simulink model "Simple_4Quad_payload_10_2017a"  (R2017a)
settings: Solver=ode45  StartTime=0.0  StopTime=100  FixedStep=0.001  RelTol=1e-3
InitFcn:
  | Simple_4Quad_payload_10_const
values from neighbouring files (symbols this model uses):
  All_rho = [d1 0 0 ... (first row only)    [Colab_4Quad_model_01_const.m]    (also in Colab_4Quad_model_02_const.m; Simple_4Quad_payload_04_const.m; Simple_4Quad_payload_05_const.m; Simple_4Quad_payload_06_const.m)
  alpha_chatt = 0.1    [Simple_4Quad_payload_09_const.m]    (also in Simple_4Quad_payload_10_const.m = 0.001; Simple_4Quad_payload_11_const.m = 0.01; Simple_4Quad_payload_12_const.m = 0.01)
  alphaTF = 0.1    [Simple_4Quad_payload_08_const.m]    (also in Simple_4Quad_payload_09_const.m = 0.5; Simple_4Quad_payload_10_const.m = 1; Simple_4Quad_payload_11_const.m = 0.5; Simple_4Quad_payload_12_const.m = 10)
  B_ob = [zeros(3);eye(3)]    [Simple_4Quad_payload_04_const.m]    (also in Simple_4Quad_payload_05_const.m; Simple_4Quad_payload_06_const.m; Simple_4Quad_payload_07_const.m; Simple_4Quad_payload_08_const.m)
  BBT_inv = ((B'*B)^(-1))*B'    [Simple_2Quad_payload_03_const.m]    (also in Simple_4Quad_payload_04_const.m = ((BR'*BR)^(-1))*BR'; Simple_4Quad_payload_05_const.m = ((BR'*BR)^(-1))*BR'; Simple_4Quad_payload_06_const.m = ((BR'*BR)^(-1))*BR'; Simple_4Quad_payload_07_const.m = ((BR'*BR)^(-1))*BR')
  BBT_invp = ((BRp'*BRp)^(-1))*BRp'    [Simple_4Quad_payload_10_const.m]    (also in Simple_4Quad_payload_11_const.m; Simple_4Quad_payload_12_const.m)
  BR = 1e0*eye(n)    [Simple_4Quad_payload_04_const.m]    (also in Simple_4Quad_payload_05_const.m; Simple_4Quad_payload_06_const.m; Simple_4Quad_payload_07_const.m; Simple_4Quad_payload_08_const.m)
  BRp = 1e0*eye(np)    [Simple_4Quad_payload_10_const.m]    (also in Simple_4Quad_payload_11_const.m; Simple_4Quad_payload_12_const.m)
  C_ob = [eye(3) zeros(3)]    [Simple_4Quad_payload_04_const.m]    (also in Simple_4Quad_payload_05_const.m; Simple_4Quad_payload_06_const.m; Simple_4Quad_payload_07_const.m; Simple_4Quad_payload_08_const.m)
  cons_sld = 0.001    [Simple_4Quad_payload_10_const.m]    (also in Simple_4Quad_payload_11_const.m = 0.01; Simple_4Quad_payload_12_const.m = 0.01)
  d1 = 0.25    [Colab_4Quad_model_01_const.m]    (also in Colab_4Quad_model_02_const.m = 0.5; Simple_4Quad_payload_01_const.m = 1; Simple_4Quad_payload_02_const.m = 1; Simple_4Quad_payload_03_const.m = 1)
  d2 = 0.25    [Colab_4Quad_model_01_const.m]    (also in Colab_4Quad_model_02_const.m = 0.5; Simple_4Quad_payload_01_const.m = 1; Simple_4Quad_payload_02_const.m = 1; Simple_4Quad_payload_03_const.m = 1)
  Des_rel_dist = 2    [Simple_4Quad_payload_01_const.m]    (also in Simple_4Quad_payload_02_const.m = 4; Simple_4Quad_payload_03_const.m = 4; Simple_4Quad_payload_04_const.m; Simple_4Quad_payload_05_const.m)
  g = 9.81    [Colab_4Quad_model_01_const.m]    (also in Colab_4Quad_model_02_const.m; Simple_2Quad_payload_01_const.m; Simple_2Quad_payload_02_const.m; Simple_2Quad_payload_03_const.m)
  gamma_0 = 1e-0*diag([1e-3;1e-0])    [Simple_2Quad_payload_03_const.m]    (also in Simple_4Quad_payload_04_const.m = 1e-0*diag([1e-6*ones(3,1);1e-0*ones(3,1)]); Simple_4Quad_payload_05_const.m = 1e-1*diag([1e-6*ones(3,1);1e-0*ones(3,1)]); Simple_4Quad_payload_06_const.m = 1e-0*diag([1e-6*ones(3,1);1e-0*ones(3,1)]); Simple_4Quad_payload_07_const.m = 1e-0*diag([1e-6*ones(3,1);1e-0*ones(3,1)]))
  gamma_0a = 1e-0*diag(1e-0*ones(3,1))    [Simple_4Quad_payload_10_const.m]    (also in Simple_4Quad_payload_11_const.m = 1e-0*diag(1e-6*ones(3,1)))
  gamma_0L = 1e-0*diag([1e-6*ones(3,1);1e-0*ones(3,1)])    [Simple_4Quad_payload_08_const.m]    (also in Simple_4Quad_payload_09_const.m; Simple_4Quad_payload_10_const.m = 1e+0*diag([1e-3*ones(3,1);1e-3*ones(3,1)]); Simple_4Quad_payload_11_const.m = 1e+0*diag([1e-3*ones(3,1);1e-3*ones(3,1)]); Simple_4Quad_payload_12_const.m = 1e+2*diag(1e-4*ones(3,1)))
  gamma_0p = 1e-0*diag(1e-3*ones(3,1))    [Simple_4Quad_payload_10_const.m]    (also in Simple_4Quad_payload_11_const.m = 1e-0*diag(1e-6*ones(3,1)))
  gamma_0r = 1e-0*diag(1e-3*ones(3,1))    [Simple_4Quad_payload_10_const.m]    (also in Simple_4Quad_payload_11_const.m = 1e-0*diag(1e-6*ones(3,1)); Simple_4Quad_payload_12_const.m = 1e+3*diag(1e-0*ones(3,1)))
  gamma_0v = 1e-0*diag([1e-0*ones(3,1);1e-0*ones(3,1)])    [Simple_4Quad_payload_08_const.m]    (also in Simple_4Quad_payload_09_const.m = 1e-0*diag([1e-6*ones(3,1);1e-6*ones(3,1)]); Simple_4Quad_payload_10_const.m = 1e+0*diag(1e-0*ones(3,1)); Simple_4Quad_payload_11_const.m = 1e+0*diag(1e-0*ones(3,1)); Simple_4Quad_payload_12_const.m = 1e+3*diag(1e-0*ones(3,1)))
  gamma_1 = 1e+2*diag([1e-3;1e-0])    [Simple_2Quad_payload_03_const.m]    (also in Simple_4Quad_payload_04_const.m = 1e+2*diag([1e-6*ones(3,1);1e-0*ones(3,1)]); Simple_4Quad_payload_05_const.m = 1e+2*diag([1e-6*ones(3,1);1e-0*ones(3,1)]); Simple_4Quad_payload_06_const.m = 1e+3*diag([1e-6*ones(3,1);1e-0*ones(3,1)]); Simple_4Quad_payload_07_const.m = 1e+3*diag([1e-6*ones(3,1);1e-0*ones(3,1)]))
  gamma_1a = 1e+0*diag(1e-0*ones(3,1))    [Simple_4Quad_payload_10_const.m]    (also in Simple_4Quad_payload_11_const.m = 1e+0*diag(1e-6*ones(3,1)))
  gamma_1L = 1e+3*diag([1e-6*ones(3,1);1e-0*ones(3,1)])    [Simple_4Quad_payload_08_const.m]    (also in Simple_4Quad_payload_09_const.m = 1e+2*diag([1e-6*ones(3,1);1e-0*ones(3,1)]); Simple_4Quad_payload_10_const.m = 1e+1*diag([1e-3*ones(3,1);1e-3*ones(3,1)]); Simple_4Quad_payload_11_const.m = 1e+0*diag([1e-3*ones(3,1);1e-3*ones(3,1)]); Simple_4Quad_payload_12_const.m = 1e+2*diag(1e-4*ones(3,1)))
  gamma_1p = 1e+0*diag(1e-3*ones(3,1))    [Simple_4Quad_payload_10_const.m]    (also in Simple_4Quad_payload_11_const.m = 1e+0*diag(1e-6*ones(3,1)))
  gamma_1r = 1e+0*diag(1e-3*ones(3,1))    [Simple_4Quad_payload_10_const.m]    (also in Simple_4Quad_payload_11_const.m = 1e+0*diag(1e-6*ones(3,1)); Simple_4Quad_payload_12_const.m = 1e+3*diag(1e-0*ones(3,1)))
  gamma_1v = 1e+3*diag([1e-0*ones(3,1);1e-0*ones(3,1)])    [Simple_4Quad_payload_08_const.m]    (also in Simple_4Quad_payload_09_const.m = 1e+2*diag([1e-6*ones(3,1);1e-6*ones(3,1)]); Simple_4Quad_payload_10_const.m = 1e+0*diag(1e-0*ones(3,1)); Simple_4Quad_payload_11_const.m = 1e+0*diag(1e-0*ones(3,1)); Simple_4Quad_payload_12_const.m = 1e+3*diag(1e-0*ones(3,1)))
  Ix = 0.166667    [Colab_4Quad_model_01_const.m]    (also in Colab_4Quad_model_02_const.m = 0.02; Simple_4Quad_payload_01_const.m = 1; Simple_4Quad_payload_02_const.m = 1; Simple_4Quad_payload_03_const.m = 1)
  Iy = 0.166667    [Colab_4Quad_model_01_const.m]    (also in Colab_4Quad_model_02_const.m = 0.02; Simple_4Quad_payload_01_const.m = 1; Simple_4Quad_payload_02_const.m = 1; Simple_4Quad_payload_03_const.m = 1)
  Iz = 0.166667    [Colab_4Quad_model_01_const.m]    (also in Colab_4Quad_model_02_const.m = 0.02; Simple_4Quad_payload_01_const.m = 1; Simple_4Quad_payload_02_const.m = 1; Simple_4Quad_payload_03_const.m = 1)
  Jo = diag([Ix;Iy;Iz])    [Colab_4Quad_model_01_const.m]    (also in Colab_4Quad_model_02_const.m; Simple_4Quad_payload_04_const.m; Simple_4Quad_payload_05_const.m; Simple_4Quad_payload_06_const.m)
  Jq = diag([0.0291 0.0291 0.0552])    [Colab_4Quad_model_01_const.m]    (also in Colab_4Quad_model_02_const.m = diag([0.03 0.03 0.06]); Simple_4Quad_payload_03_const.m = 1.2416e-3 * diag([1 1 2]); Simple_4Quad_payload_04_const.m = 1 * diag([1 1 2]); Simple_4Quad_payload_05_const.m = 1 * diag([1 1 2]))
  k1 = 1    [Simple_2Quad_payload_03_const.m]    (also in Simple_4Quad_payload_04_const.m; Simple_4Quad_payload_05_const.m; Simple_4Quad_payload_06_const.m; Simple_4Quad_payload_07_const.m)
  k2 = 0.1    [Simple_2Quad_payload_03_const.m]    (also in Simple_4Quad_payload_04_const.m; Simple_4Quad_payload_05_const.m; Simple_4Quad_payload_06_const.m; Simple_4Quad_payload_07_const.m)
  l = 3.1819    [Colab_4Quad_model_01_const.m]    (also in Colab_4Quad_model_02_const.m = 3; Simple_2Quad_payload_04_const.m = 1; Simple_4Quad_payload_01_const.m = 1; Simple_4Quad_payload_02_const.m = 2)
  m = 1.5    [Colab_4Quad_model_01_const.m]    (also in Colab_4Quad_model_02_const.m; Simple_2Quad_payload_04_const.m = 1; Simple_4Quad_payload_01_const.m = 1; Simple_4Quad_payload_02_const.m = 1)
  M = 1.0    (= 1)    [Colab_4Quad_model_01_const.m]    (also in Colab_4Quad_model_02_const.m; Simple_2Quad_payload_01_const.m; Simple_2Quad_payload_02_const.m; Simple_2Quad_payload_03_const.m)
  n = 2    [Simple_2Quad_payload_03_const.m]    (also in Simple_4Quad_payload_03_const.m = 6; Simple_4Quad_payload_04_const.m = 6; Simple_4Quad_payload_05_const.m = 6; Simple_4Quad_payload_06_const.m = 6)
  noise_var_RelAcc = 0e-6    (= 0)    [Simple_4Quad_payload_07_const.m]    (also in Simple_4Quad_payload_08_const.m; Simple_4Quad_payload_09_const.m; Simple_4Quad_payload_10_const.m; Simple_4Quad_payload_11_const.m)
  noise_var_RelPos = 0e-6    (= 0)    [Simple_4Quad_payload_07_const.m]    (also in Simple_4Quad_payload_08_const.m; Simple_4Quad_payload_09_const.m; Simple_4Quad_payload_10_const.m; Simple_4Quad_payload_11_const.m)
  np = 3    [Simple_4Quad_payload_10_const.m]    (also in Simple_4Quad_payload_11_const.m; Simple_4Quad_payload_12_const.m; constant_CAMFC2_Quad_New_02_Payload_01.m = 6)
  Q_ob = var_u_ob * eye(6)    [Simple_4Quad_payload_04_const.m]    (also in Simple_4Quad_payload_05_const.m; Simple_4Quad_payload_06_const.m; Simple_4Quad_payload_07_const.m; Simple_4Quad_payload_08_const.m)
  Qa = 1e-0*eye(np)    [Simple_4Quad_payload_10_const.m]    (also in Simple_4Quad_payload_11_const.m)
  QL = 1e-0*eye(n)    [Simple_4Quad_payload_08_const.m]    (also in Simple_4Quad_payload_09_const.m; Simple_4Quad_payload_10_const.m; Simple_4Quad_payload_11_const.m = 1e-2*eye(n); Simple_4Quad_payload_12_const.m = 1e-0*eye(np))
  Qp = 1e-0*eye(np)    [Simple_4Quad_payload_10_const.m]    (also in Simple_4Quad_payload_11_const.m = 1e-2*eye(np))
  QR = 1e-0*eye(n)    [Simple_4Quad_payload_04_const.m]    (also in Simple_4Quad_payload_05_const.m = 1e-1*eye(n); Simple_4Quad_payload_06_const.m; Simple_4Quad_payload_07_const.m; Simple_4Quad_payload_08_const.m)
  Qr = 1e-0*eye(np)    [Simple_4Quad_payload_10_const.m]    (also in Simple_4Quad_payload_11_const.m; Simple_4Quad_payload_12_const.m)
  Qv = 1e-0*eye(n)    [Simple_4Quad_payload_08_const.m]    (also in Simple_4Quad_payload_09_const.m; Simple_4Quad_payload_10_const.m = 1e-0*eye(np); Simple_4Quad_payload_11_const.m = 1e-2*eye(np); Simple_4Quad_payload_12_const.m = 1e-0*eye(np))
  R = 1e+0*eye(n)    [Simple_2Quad_payload_03_const.m]    (also in Simple_4Quad_payload_04_const.m = 1e+0*eye(m); Simple_4Quad_payload_05_const.m = 1e+0*eye(m); Simple_4Quad_payload_06_const.m; Simple_4Quad_payload_07_const.m)
  R_ob = var_y_ob * eye(3)    [Simple_4Quad_payload_04_const.m]    (also in Simple_4Quad_payload_05_const.m; Simple_4Quad_payload_06_const.m; Simple_4Quad_payload_07_const.m; Simple_4Quad_payload_08_const.m)
  rho_0 = 1e-0    (= 1)    [Simple_2Quad_payload_03_const.m]    (also in Simple_4Quad_payload_04_const.m; Simple_4Quad_payload_05_const.m = 0.1; Simple_4Quad_payload_06_const.m; Simple_4Quad_payload_07_const.m)
  rho_0a = 1e-0    (= 1)    [Simple_4Quad_payload_10_const.m]    (also in Simple_4Quad_payload_11_const.m)
  rho_0L = 1e-0    (= 1)    [Simple_4Quad_payload_08_const.m]    (also in Simple_4Quad_payload_09_const.m; Simple_4Quad_payload_10_const.m; Simple_4Quad_payload_11_const.m; Simple_4Quad_payload_12_const.m)
  rho_0p = 1e-0    (= 1)    [Simple_4Quad_payload_10_const.m]    (also in Simple_4Quad_payload_11_const.m)
  rho_0r = 1e-0    (= 1)    [Simple_4Quad_payload_10_const.m]    (also in Simple_4Quad_payload_11_const.m; Simple_4Quad_payload_12_const.m = 0.001)
  rho_0v = 1e-1    (= 0.1)    [Simple_4Quad_payload_08_const.m]    (also in Simple_4Quad_payload_09_const.m = 1; Simple_4Quad_payload_10_const.m = 1; Simple_4Quad_payload_11_const.m = 1; Simple_4Quad_payload_12_const.m = 1)
  rho_1 = 1e-0    (= 1)    [Simple_2Quad_payload_03_const.m]    (also in Simple_4Quad_payload_04_const.m; Simple_4Quad_payload_05_const.m; Simple_4Quad_payload_06_const.m; Simple_4Quad_payload_07_const.m)
  rho_1a = 1e-0    (= 1)    [Simple_4Quad_payload_10_const.m]    (also in Simple_4Quad_payload_11_const.m)
  rho_1L = 1e-0    (= 1)    [Simple_4Quad_payload_08_const.m]    (also in Simple_4Quad_payload_09_const.m; Simple_4Quad_payload_10_const.m; Simple_4Quad_payload_11_const.m; Simple_4Quad_payload_12_const.m)
  rho_1p = 1e-0    (= 1)    [Simple_4Quad_payload_10_const.m]    (also in Simple_4Quad_payload_11_const.m)
  rho_1r = 1e-0    (= 1)    [Simple_4Quad_payload_10_const.m]    (also in Simple_4Quad_payload_11_const.m; Simple_4Quad_payload_12_const.m)
  rho_1v = 1e-0    (= 1)    [Simple_4Quad_payload_08_const.m]    (also in Simple_4Quad_payload_09_const.m; Simple_4Quad_payload_10_const.m; Simple_4Quad_payload_11_const.m; Simple_4Quad_payload_12_const.m)
  Rp = 1e+0*eye(np)    [Simple_4Quad_payload_10_const.m]    (also in Simple_4Quad_payload_11_const.m; Simple_4Quad_payload_12_const.m)
  xo_init = 0    [Simple_4Quad_payload_10_const.m]    (also in Simple_4Quad_payload_11_const.m; Simple_4Quad_payload_12_const.m)
  yo_init = 0    [Simple_4Quad_payload_10_const.m]    (also in Simple_4Quad_payload_11_const.m; Simple_4Quad_payload_12_const.m)
  zo_init = 0    [Simple_4Quad_payload_10_const.m]    (also in Simple_4Quad_payload_11_const.m; Simple_4Quad_payload_12_const.m)
libraries: simulink x2
(part 4 of 5)

== matlab function Simple_4Quad_payload_10_2017a/Controllers and Observers/Controller and Observer - Agent4/Rotational #4/Differentiator/Sliding differentiator ==
  data: u output; u1 input; e input; n parameter; k1 parameter; cons_sld parameter
function u = fcn(u1,e,n,k1,cons_sld)

b=k1;

ABS = zeros(n,1);
for i=1:n
    if e(i)>0
        ABS(i) = e(i);
    else
        ABS(i) = -e(i);
    end
end
SGN = e ./ (ABS + cons_sld);

u = u1 - b*(ABS.^0.5).*SGN;

end

== matlab function Simple_4Quad_payload_10_2017a/Controllers and Observers/Controller and Observer - Agent4/Rotational #4/Differentiator/Sliding differentiator1 ==
  data: Du1 output; e input; n parameter; k2 parameter; cons_sld parameter
function Du1 = fcn(e,n,k2,cons_sld)

a=k2;

ABS = zeros(n,1);
for i=1:n
    if e(i)>0
        ABS(i) = e(i);
    else
        ABS(i) = -e(i);
    end
end
SGN = e ./ (ABS + cons_sld);

Du1 = - a*SGN;

end

== matlab function Simple_4Quad_payload_10_2017a/Controllers and Observers/Controller and Observer - Agent4/Rotational #4/g-Estimator ==
  data: sigma input; g_hat input; P input; rho_1 parameter; gamma_1 parameter; Dg_hat output
function Dg_hat = fcn(sigma,g_hat,P,rho_1,gamma_1)

Dg_hat = - gamma_1 * P * sigma - rho_1 * gamma_1 * g_hat;

end

== matlab function Simple_4Quad_payload_10_2017a/Controllers and Observers/Controller and Observer - Agent4/Rotational #4/g-Estimator1 ==
  data: sigma input; x input; P input; rho_0 parameter; gamma_0 parameter; Da_hat output; a_hat input
function Da_hat = fcn(sigma,x,P,rho_0,gamma_0,a_hat)

DVa_hat = - gamma_0 * P * diag(sigma) * (x - sigma) - rho_0 * gamma_0 * diag(a_hat);

Da_hat = diag(DVa_hat);

end

== matlab function Simple_4Quad_payload_10_2017a/Controllers and Observers/Controller and Observer - Agent4/Rotational #4/main ==
  data: sigma input; zeta input; u output; Dy_d input; R parameter; P input; a_hat input; BR parameter; g_hat input; x input; QR parameter; BBT_inv parameter; n parameter
function u = fcn(sigma,zeta,Dy_d,R,P,a_hat,BR,g_hat,x,QR,BBT_inv,n)

u1 = (1/2) * R * BR' * P * sigma;
u2 = BBT_inv * (Dy_d - a_hat*x + (eye(n) + 2*(((P)^(-1)*QR)) + a_hat)*sigma - g_hat - zeta) - (3/4) * R * BR' * P * sigma;

u = u1 + u2;

end

== matlab function Simple_4Quad_payload_10_2017a/Controllers and Observers/Controller and Observer - Agent4/Rotational #4/variable change ==
  data: X input; Xd input; x_mod output; u input; xd_mod output; e_mod output
function [x_mod,xd_mod,e_mod] = fcn(X,Xd,u)

x_mod = X;

xd_mod = [Xd;u(1:3)];

e_mod = xd_mod - x_mod;


end

== matlab function Simple_4Quad_payload_10_2017a/Controllers and Observers/Controlelr and Observer - Agent3/Observer3/Kalman_Filter3 ==
  data: P_ob input; DP_ob output; xhat_ob input; Dxhat_ob output; Q_ob parameter; R_ob parameter; C_ob parameter; B_ob parameter; wo input; Dwo input; Rel_Posi_local input; Rel_Acci_local input; Agent_Num input; All_rho parameter; l parameter
function [DP_ob,Dxhat_ob] = fcn(P_ob,xhat_ob,Q_ob, R_ob, C_ob, B_ob,wo,Dwo,Rel_Posi_local,Rel_Acci_local,Agent_Num,All_rho,l)

rhoi = All_rho(Agent_Num,:)';

wo_skew = [...
    0 -wo(3) wo(2);
    wo(3) 0 -wo(1);
    -wo(2) wo(1) 0];

Dwo_skew = [...
    0 -Dwo(3) Dwo(2);
    Dwo(3) 0 -Dwo(1);
    -Dwo(2) Dwo(1) 0];

A1_ob = wo_skew * wo_skew + Dwo_skew;
A2_ob = 2*wo_skew;

A_ob = [zeros(3) eye(3);
    -A1_ob -A2_ob];

y_ob = (1/l) * ( Rel_Posi_local - rhoi );
u_ob = (1/l) * ( Rel_Acci_local - A1_ob*rhoi );

DP_ob = A_ob'*P_ob + P_ob*A_ob - P_ob*C_ob'*R_ob*C_ob*P_ob + Q_ob;
K_ob = P_ob * C_ob' * R_ob;
Dxhat_ob = A_ob*xhat_ob + B_ob*u_ob + K_ob*(y_ob - C_ob*xhat_ob);

end

== matlab function Simple_4Quad_payload_10_2017a/Controllers and Observers/Controlelr and Observer - Agent3/Observer3/Observer_Finalization3 ==
  data: xhati input; qhati output; Dqhati output
function [qhati,Dqhati] = fcn(xhati)

qhati = xhati(1:3);
Dqhati = xhati(4:6);

end

== matlab function Simple_4Quad_payload_10_2017a/Controllers and Observers/Controller and Observer - Agent4/Observer4/Kalman_Filter4 ==
  data: P_ob input; DP_ob output; xhat_ob input; Dxhat_ob output; Q_ob parameter; R_ob parameter; C_ob parameter; B_ob parameter; wo input; Dwo input; Rel_Posi_local input; Rel_Acci_local input; Agent_Num input; All_rho parameter; l parameter
function [DP_ob,Dxhat_ob] = fcn(P_ob,xhat_ob,Q_ob, R_ob, C_ob, B_ob,wo,Dwo,Rel_Posi_local,Rel_Acci_local,Agent_Num,All_rho,l)

rhoi = All_rho(Agent_Num,:)';

wo_skew = [...
    0 -wo(3) wo(2);
    wo(3) 0 -wo(1);
    -wo(2) wo(1) 0];

Dwo_skew = [...
    0 -Dwo(3) Dwo(2);
    Dwo(3) 0 -Dwo(1);
    -Dwo(2) Dwo(1) 0];

A1_ob = wo_skew * wo_skew + Dwo_skew;
A2_ob = 2*wo_skew;

A_ob = [zeros(3) eye(3);
    -A1_ob -A2_ob];

y_ob = (1/l) * ( Rel_Posi_local - rhoi );
u_ob = (1/l) * ( Rel_Acci_local - A1_ob*rhoi );

DP_ob = A_ob'*P_ob + P_ob*A_ob - P_ob*C_ob'*R_ob*C_ob*P_ob + Q_ob;
K_ob = P_ob * C_ob' * R_ob;
Dxhat_ob = A_ob*xhat_ob + B_ob*u_ob + K_ob*(y_ob - C_ob*xhat_ob);

end

== matlab function Simple_4Quad_payload_10_2017a/Controllers and Observers/Controller and Observer - Agent4/Observer4/Observer_Finalization4 ==
  data: xhati input; qhati output; Dqhati output
function [qhati,Dqhati] = fcn(xhati)

qhati = xhati(1:3);
Dqhati = xhati(4:6);

end

== matlab function Simple_4Quad_payload_10_2017a/Relative measurements/Relative position measurements in payload local frame ==
  data: PHI input; Rel_Pos_local1 output; ro input; r1 input; r2 input; r3 input; r4 input; Rel_Pos_local2 output; Rel_Pos_local3 output; Rel_Pos_local4 output
function [Rel_Pos_local1,Rel_Pos_local2,Rel_Pos_local3,Rel_Pos_local4] = fcn(PHI,ro,r1,r2,r3,r4)

phi = PHI(1);
theta = PHI(2);
psi = PHI(3);

Ro = [cos(psi)*cos(theta) cos(psi)*sin(theta)*sin(phi)-sin(psi)*cos(phi) cos(psi)*sin(theta)*cos(phi)+sin(psi)*sin(phi);
    sin(psi)*cos(theta) sin(psi)*sin(theta)*sin(phi)+cos(psi)*cos(phi) sin(psi)*sin(theta)*cos(phi)-cos(psi)*sin(phi);
    -sin(theta) cos(theta)*sin(phi) cos(theta)*cos(phi)];

Rel_Pos_local1 = Ro' * (r1 - ro);
Rel_Pos_local2 = Ro' * (r2 - ro);
Rel_Pos_local3 = Ro' * (r3 - ro);
Rel_Pos_local4 = Ro' * (r4 - ro);

end

== matlab function Simple_4Quad_payload_10_2017a/Dynamic model of the entire system/Drone absolute position computation ==
  data: q1 input; r1 output; r2 output; r3 output; r4 output; q2 input; q3 input; q4 input; All_rho parameter; l parameter; ro input; PHI input
function [r1,r2,r3,r4] = fcn(q1,q2,q3,q4,All_rho, l,ro,PHI)

rho1 = All_rho(1,:)';
rho2 = All_rho(2,:)';
rho3 = All_rho(3,:)';
rho4 = All_rho(4,:)';

phi = PHI(1);
theta = PHI(2);
psi = PHI(3);

Ro = [cos(psi)*cos(theta) cos(psi)*sin(theta)*sin(phi)-sin(psi)*cos(phi) cos(psi)*sin(theta)*cos(phi)+sin(psi)*sin(phi);
    sin(psi)*cos(theta) sin(psi)*sin(theta)*sin(phi)+cos(psi)*cos(phi) sin(psi)*sin(theta)*cos(phi)-cos(psi)*sin(phi);
    -sin(theta) cos(theta)*sin(phi) cos(theta)*cos(phi)];

r1 = ro + Ro*rho1 - l*q1;
r2 = ro + Ro*rho2 - l*q2;
r3 = ro + Ro*rho3 - l*q3;
r4 = ro + Ro*rho4 - l*q4;

end

== matlab function Simple_4Quad_payload_10_2017a/Relative measurements/Relative acceleration measurements in payload local frame ==
  data: PHI input; Rel_Acc_local1 output; DDro input; DDr1 input; DDr2 input; DDr3 input; DDr4 input; Rel_Acc_local2 output; Rel_Acc_local3 output; Rel_Acc_local4 output
function [Rel_Acc_local1,Rel_Acc_local2,Rel_Acc_local3,Rel_Acc_local4] = fcn(PHI,DDro,DDr1,DDr2,DDr3,DDr4)

phi = PHI(1);
theta = PHI(2);
psi = PHI(3);

Ro = [cos(psi)*cos(theta) cos(psi)*sin(theta)*sin(phi)-sin(psi)*cos(phi) cos(psi)*sin(theta)*cos(phi)+sin(psi)*sin(phi);
    sin(psi)*cos(theta) sin(psi)*sin(theta)*sin(phi)+cos(psi)*cos(phi) sin(psi)*sin(theta)*cos(phi)-cos(psi)*sin(phi);
    -sin(theta) cos(theta)*sin(phi) cos(theta)*cos(phi)];

Rel_Acc_local1 = Ro' * (DDr1 - DDro);
Rel_Acc_local2 = Ro' * (DDr2 - DDro);
Rel_Acc_local3 = Ro' * (DDr3 - DDro);
Rel_Acc_local4 = Ro' * (DDr4 - DDro);

end

== matlab function Simple_4Quad_payload_10_2017a/Dynamic model of the entire system/Drone absolute acceleration computation ==
  data: q1 input; DDr1 output; DDr2 output; DDr3 output; DDr4 output; q2 input; q3 input; q4 input; wi1 input; wi2 input; wi3 input; wi4 input; Dwi1 input; Dwi2 input; Dwi3 input; Dwi4 input; All_rho parameter; l parameter; DDro input; PHI input; wo input; Dwo input
function [DDr1,DDr2,DDr3,DDr4] = fcn(q1,q2,q3,q4,wi1,wi2,wi3,wi4,Dwi1,Dwi2,Dwi3,Dwi4,All_rho, l,DDro,PHI,wo,Dwo)

rho1 = All_rho(1,:)';
rho2 = All_rho(2,:)';
rho3 = All_rho(3,:)';
rho4 = All_rho(4,:)';

phi = PHI(1);
theta = PHI(2);
psi = PHI(3);

wo_skew = [...
    0 -wo(3) wo(2);
    wo(3) 0 -wo(1);
    -wo(2) wo(1) 0];

Dwo_skew = [...
    0 -Dwo(3) Dwo(2);
    Dwo(3) 0 -Dwo(1);
    -Dwo(2) Dwo(1) 0];

wi1_skew = [...
    0 -wi1(3) wi1(2);
    wi1(3) 0 -wi1(1);
    -wi1(2) wi1(1) 0];

Dwi1_skew = [...
    0 -Dwi1(3) Dwi1(2);
    Dwi1(3) 0 -Dwi1(1);
    -Dwi1(2) Dwi1(1) 0];

wi2_skew = [...
    0 -wi2(3) wi2(2);
    wi2(3) 0 -wi2(1);
    -wi2(2) wi2(1) 0];

Dwi2_skew = [...
    0 -Dwi2(3) Dwi2(2);
    Dwi2(3) 0 -Dwi2(1);
    -Dwi2(2) Dwi2(1) 0];

wi3_skew = [...
    0 -wi3(3) wi3(2);
    wi3(3) 0 -wi3(1);
    -wi3(2) wi3(1) 0];

Dwi3_skew = [...
    0 -Dwi3(3) Dwi3(2);
    Dwi3(3) 0 -Dwi3(1);
    -Dwi3(2) Dwi3(1) 0];

wi4_skew = [...
    0 -wi4(3) wi4(2);
    wi4(3) 0 -wi4(1);
    -wi4(2) wi4(1) 0];

Dwi4_skew = [...
    0 -Dwi4(3) Dwi4(2);
    Dwi4(3) 0 -Dwi4(1);
    -Dwi4(2) Dwi4(1) 0];


Ro = [cos(psi)*cos(theta) cos(psi)*sin(theta)*sin(phi)-sin(psi)*cos(phi) cos(psi)*sin(theta)*cos(phi)+sin(psi)*sin(phi);
    sin(psi)*cos(theta) sin(psi)*sin(theta)*sin(phi)+cos(psi)*cos(phi) sin(psi)*sin(theta)*cos(phi)-cos(psi)*sin(phi);
    -sin(theta) cos(theta)*sin(phi) cos(theta)*cos(phi)];

DDr1 = DDro + Ro*wo_skew*wo_skew*rho1 + Ro*Dwo_skew*rho1 - l*wi1_skew*wi1_skew*q1 - l*Dwi1_skew*q1;
DDr2 = DDro + Ro*wo_skew*wo_skew*rho2 + Ro*Dwo_skew*rho2 - l*wi2_skew*wi2_skew*q2 - l*Dwi2_skew*q2;
DDr3 = DDro + Ro*wo_skew*wo_skew*rho3 + Ro*Dwo_skew*rho3 - l*wi3_skew*wi3_skew*q3 - l*Dwi3_skew*q3;
DDr4 = DDro + Ro*wo_skew*wo_skew*rho4 + Ro*Dwo_skew*rho4 - l*wi4_skew*wi4_skew*q4 - l*Dwi4_skew*q4;


end

== matlab function Simple_4Quad_payload_10_2017a/Controllers and Observers/Cotnroller and Observer - Agent1 /Rotational #1/output definition ==
  data: u input; ur output
function ur = fcn(u)

ur = u(4:6);

end

== matlab function Simple_4Quad_payload_10_2017a/Controllers and Observers/Controller and Observer - Agent2/Rotational #2/output definition ==
  data: u input; ur output
function ur = fcn(u)

ur = u(4:6);

end

== matlab function Simple_4Quad_payload_10_2017a/Controllers and Observers/Cotnroller and Observer - Agent1 /Rotational #1/CARE ==
  data: P input; a_hat input; BR parameter; R parameter; DP output; QR parameter
function DP = fcn(P,a_hat,BR,R,QR)

DP = a_hat*P + P*a_hat' - P*BR*R*BR'*P + 2*QR;

end

== matlab function Simple_4Quad_payload_10_2017a/Controllers and Observers/Controlelr and Observer - Agent3/Rotational #3/output definition ==
  data: u input; ur output
function ur = fcn(u)

ur = u(4:6);

end

== matlab function Simple_4Quad_payload_10_2017a/Controllers and Observers/Controller and Observer - Agent4/Rotational #4/output definition ==
  data: u input; ur output
function ur = fcn(u)

ur = u(4:6);

end

== matlab function Simple_4Quad_payload_10_2017a/Dynamic model of the entire system/Control inputs from Q1/Controller Interpreter #1 ==
  data: UTi input; qi input; PHIi input; Ui_local_paral output; Ui_local_perpn output
function [Ui_local_paral,Ui_local_perpn] = fcn(UTi,qi,PHIi)

phi_i = PHIi(1);
theta_i = PHIi(2);
psi_i = PHIi(3);

Ri = [cos(psi_i)*cos(theta_i) cos(psi_i)*sin(theta_i)*sin(phi_i)-sin(psi_i)*cos(phi_i) cos(psi_i)*sin(theta_i)*cos(phi_i)+sin(psi_i)*sin(phi_i);
    sin(psi_i)*cos(theta_i) sin(psi_i)*sin(theta_i)*sin(phi_i)+cos(psi_i)*cos(phi_i) sin(psi_i)*sin(theta_i)*cos(phi_i)-cos(psi_i)*sin(phi_i);
    -sin(theta_i) cos(theta_i)*sin(phi_i) cos(theta_i)*cos(phi_i)]; 

Ui_local_paral = (qi*qi') * (Ri * UTi);
Ui_local_perpn = (eye(3) - qi*qi') * (Ri * UTi);


end

== matlab function Simple_4Quad_payload_10_2017a/Controllers and Observers/Cotnroller and Observer - Agent1 /Link #1/CARE ==
  data: P input; a_hat input; BR parameter; R parameter; DP output; QL parameter
function DP = fcn(P,a_hat,BR,R,QL)

DP = a_hat*P + P*a_hat' - P*BR*R*BR'*P + 2*QL;

end

== matlab function Simple_4Quad_payload_10_2017a/Controllers and Observers/Cotnroller and Observer - Agent1 /Link #1/Differentiator/Sliding differentiator ==
  data: u output; u1 input; e input; n parameter; k1 parameter; cons_sld parameter
function u = fcn(u1,e,n,k1,cons_sld)

b=k1;

ABS = zeros(n,1);
for i=1:n
    if e(i)>0
        ABS(i) = e(i);
    else
        ABS(i) = -e(i);
    end
end
SGN = e ./ (ABS + cons_sld);

u = u1 - b*(ABS.^0.5).*SGN;

end

== matlab function Simple_4Quad_payload_10_2017a/Controllers and Observers/Cotnroller and Observer - Agent1 /Link #1/Differentiator/Sliding differentiator1 ==
  data: Du1 output; e input; n parameter; k2 parameter; cons_sld parameter
function Du1 = fcn(e,n,k2,cons_sld)

a=k2;

ABS = zeros(n,1);
for i=1:n
    if e(i)>0
        ABS(i) = e(i);
    else
        ABS(i) = -e(i);
    end
end
SGN = e ./ (ABS + cons_sld);

Du1 = - a*SGN;

end

== matlab function Simple_4Quad_payload_10_2017a/Dynamic model of the entire system/Control inputs from Q2/Controller Interpreter #2 ==
  data: UTi input; qi input; PHIi input; Ui_local_paral output; Ui_local_perpn output
function [Ui_local_paral,Ui_local_perpn] = fcn(UTi,qi,PHIi)

phi_i = PHIi(1);
theta_i = PHIi(2);
psi_i = PHIi(3);

Ri = [cos(psi_i)*cos(theta_i) cos(psi_i)*sin(theta_i)*sin(phi_i)-sin(psi_i)*cos(phi_i) cos(psi_i)*sin(theta_i)*cos(phi_i)+sin(psi_i)*sin(phi_i);
    sin(psi_i)*cos(theta_i) sin(psi_i)*sin(theta_i)*sin(phi_i)+cos(psi_i)*cos(phi_i) sin(psi_i)*sin(theta_i)*cos(phi_i)-cos(psi_i)*sin(phi_i);
    -sin(theta_i) cos(theta_i)*sin(phi_i) cos(theta_i)*cos(phi_i)]; 

Ui_local_paral = (qi*qi') * (Ri * UTi);
Ui_local_perpn = (eye(3) - qi*qi') * (Ri * UTi);


end

== matlab function Simple_4Quad_payload_10_2017a/Dynamic model of the entire system/Control inputs from Q3/Controller Interpreter #3 ==
  data: UTi input; qi input; PHIi input; Ui_local_paral output; Ui_local_perpn output
function [Ui_local_paral,Ui_local_perpn] = fcn(UTi,qi,PHIi)

phi_i = PHIi(1);
theta_i = PHIi(2);
psi_i = PHIi(3);

Ri = [cos(psi_i)*cos(theta_i) cos(psi_i)*sin(theta_i)*sin(phi_i)-sin(psi_i)*cos(phi_i) cos(psi_i)*sin(theta_i)*cos(phi_i)+sin(psi_i)*sin(phi_i);
    sin(psi_i)*cos(theta_i) sin(psi_i)*sin(theta_i)*sin(phi_i)+cos(psi_i)*cos(phi_i) sin(psi_i)*sin(theta_i)*cos(phi_i)-cos(psi_i)*sin(phi_i);
    -sin(theta_i) cos(theta_i)*sin(phi_i) cos(theta_i)*cos(phi_i)]; 

Ui_local_paral = (qi*qi') * (Ri * UTi);
Ui_local_perpn = (eye(3) - qi*qi') * (Ri * UTi);


end

== matlab function Simple_4Quad_payload_10_2017a/Dynamic model of the entire system/Control inputs from Q4/Controller Interpreter #4 ==
  data: UTi input; qi input; PHIi input; Ui_local_paral output; Ui_local_perpn output
function [Ui_local_paral,Ui_local_perpn] = fcn(UTi,qi,PHIi)

phi_i = PHIi(1);
theta_i = PHIi(2);
psi_i = PHIi(3);

Ri = [cos(psi_i)*cos(theta_i) cos(psi_i)*sin(theta_i)*sin(phi_i)-sin(psi_i)*cos(phi_i) cos(psi_i)*sin(theta_i)*cos(phi_i)+sin(psi_i)*sin(phi_i);
    sin(psi_i)*cos(theta_i) sin(psi_i)*sin(theta_i)*sin(phi_i)+cos(psi_i)*cos(phi_i) sin(psi_i)*sin(theta_i)*cos(phi_i)-cos(psi_i)*sin(phi_i);
    -sin(theta_i) cos(theta_i)*sin(phi_i) cos(theta_i)*cos(phi_i)]; 

Ui_local_paral = (qi*qi') * (Ri * UTi);
Ui_local_perpn = (eye(3) - qi*qi') * (Ri * UTi);


end

== matlab function Simple_4Quad_payload_10_2017a/Controllers and Observers/Cotnroller and Observer - Agent1 /Link #1/g-Estimator ==
  data: sigma input; g_hat input; P input; rho_1L parameter; gamma_1L parameter; Dg_hat output
function Dg_hat = fcn(sigma,g_hat,P,rho_1L,gamma_1L)

Dg_hat = - gamma_1L * P * sigma - rho_1L * gamma_1L * g_hat;

end

== matlab function Simple_4Quad_payload_10_2017a/Controllers and Observers/Cotnroller and Observer - Agent1 /Link #1/g-Estimator1 ==
  data: sigma input; x input; P input; rho_0L parameter; gamma_0L parameter; Da_hat output; a_hat input
function Da_hat = fcn(sigma,x,P,rho_0L,gamma_0L,a_hat)

DVa_hat = - gamma_0L * P * diag(sigma) * (x - sigma) - rho_0L * gamma_0L * diag(a_hat);

Da_hat = diag(DVa_hat);

end

== matlab function Simple_4Quad_payload_10_2017a/Controllers and Observers/Cotnroller and Observer - Agent1 /Link #1/main ==
  data: sigma input; zeta input; u output; Dy_d input; R parameter; P input; a_hat input; BR parameter; g_hat input; x input; QL parameter; BBT_inv parameter; n parameter
function u = fcn(sigma,zeta,Dy_d,R,P,a_hat,BR,g_hat,x,QL,BBT_inv,n)

u1 = (1/2) * R * BR' * P * sigma;
u2 = BBT_inv * (Dy_d - a_hat*x + (eye(n) + 2*(((P)^(-1)*QL)) + a_hat)*sigma - g_hat - zeta) - (3/4) * R * BR' * P * sigma;

u = u1 + u2;

end

== matlab function Simple_4Quad_payload_10_2017a/Controllers and Observers/Cotnroller and Observer - Agent1 /Link #1/output definition ==
  data: u input; ur output
function ur = fcn(u)

ur = u(4:6);

end

== matlab function Simple_4Quad_payload_10_2017a/Controllers and Observers/Cotnroller and Observer - Agent1 /Link #1/variable change ==
  data: X input; Xd input; x_mod output; u input; xd_mod output; e_mod output
function [x_mod,xd_mod,e_mod] = fcn(X,Xd,u)

x_mod = X;

xd_mod = [Xd;u(1:3)];

e_mod = xd_mod - x_mod;


end

== matlab function Simple_4Quad_payload_10_2017a/Controllers and Observers/Controller and Observer - Agent2/Link #2/CARE ==
  data: P input; a_hat input; BR parameter; R parameter; DP output; QL parameter
function DP = fcn(P,a_hat,BR,R,QL)

DP = a_hat*P + P*a_hat' - P*BR*R*BR'*P + 2*QL;

end

== matlab function Simple_4Quad_payload_10_2017a/Controllers and Observers/Controller and Observer - Agent2/Link #2/Differentiator/Sliding differentiator ==
  data: u output; u1 input; e input; n parameter; k1 parameter; cons_sld parameter
function u = fcn(u1,e,n,k1,cons_sld)

b=k1;

ABS = zeros(n,1);
for i=1:n
    if e(i)>0
        ABS(i) = e(i);
    else
        ABS(i) = -e(i);
    end
end
SGN = e ./ (ABS + cons_sld);

u = u1 - b*(ABS.^0.5).*SGN;

end

== matlab function Simple_4Quad_payload_10_2017a/Controllers and Observers/Controller and Observer - Agent2/Link #2/Differentiator/Sliding differentiator1 ==
  data: Du1 output; e input; n parameter; k2 parameter; cons_sld parameter
function Du1 = fcn(e,n,k2,cons_sld)

a=k2;

ABS = zeros(n,1);
for i=1:n
    if e(i)>0
        ABS(i) = e(i);
    else
        ABS(i) = -e(i);
    end
end
SGN = e ./ (ABS + cons_sld);

Du1 = - a*SGN;

end

== matlab function Simple_4Quad_payload_10_2017a/Controllers and Observers/Controller and Observer - Agent2/Link #2/g-Estimator ==
  data: sigma input; g_hat input; P input; rho_1L parameter; gamma_1L parameter; Dg_hat output
function Dg_hat = fcn(sigma,g_hat,P,rho_1L,gamma_1L)

Dg_hat = - gamma_1L * P * sigma - rho_1L * gamma_1L * g_hat;

end

== matlab function Simple_4Quad_payload_10_2017a/Controllers and Observers/Controller and Observer - Agent2/Link #2/g-Estimator1 ==
  data: sigma input; x input; P input; rho_0L parameter; gamma_0L parameter; Da_hat output; a_hat input
function Da_hat = fcn(sigma,x,P,rho_0L,gamma_0L,a_hat)

DVa_hat = - gamma_0L * P * diag(sigma) * (x - sigma) - rho_0L * gamma_0L * diag(a_hat);

Da_hat = diag(DVa_hat);

end

== matlab function Simple_4Quad_payload_10_2017a/Controllers and Observers/Controller and Observer - Agent2/Link #2/main ==
  data: sigma input; zeta input; u output; Dy_d input; R parameter; P input; a_hat input; BR parameter; g_hat input; x input; QL parameter; BBT_inv parameter; n parameter
function u = fcn(sigma,zeta,Dy_d,R,P,a_hat,BR,g_hat,x,QL,BBT_inv,n)

u1 = (1/2) * R * BR' * P * sigma;
u2 = BBT_inv * (Dy_d - a_hat*x + (eye(n) + 2*(((P)^(-1)*QL)) + a_hat)*sigma - g_hat - zeta) - (3/4) * R * BR' * P * sigma;

u = u1 + u2;

end

== matlab function Simple_4Quad_payload_10_2017a/Controllers and Observers/Controller and Observer - Agent2/Link #2/output definition ==
  data: u input; ur output
function ur = fcn(u)

ur = u(4:6);

end

== matlab function Simple_4Quad_payload_10_2017a/Controllers and Observers/Controller and Observer - Agent2/Link #2/variable change ==
  data: X input; Xd input; x_mod output; u input; xd_mod output; e_mod output
function [x_mod,xd_mod,e_mod] = fcn(X,Xd,u)

x_mod = X;

xd_mod = [Xd;u(1:3)];

e_mod = xd_mod - x_mod;


end

== matlab function Simple_4Quad_payload_10_2017a/Controllers and Observers/Controlelr and Observer - Agent3/Link #3/CARE ==
  data: P input; a_hat input; BR parameter; R parameter; DP output; QL parameter
function DP = fcn(P,a_hat,BR,R,QL)

DP = a_hat*P + P*a_hat' - P*BR*R*BR'*P + 2*QL;

end

== matlab function Simple_4Quad_payload_10_2017a/Controllers and Observers/Controlelr and Observer - Agent3/Link #3/Differentiator/Sliding differentiator ==
  data: u output; u1 input; e input; n parameter; k1 parameter; cons_sld parameter
function u = fcn(u1,e,n,k1,cons_sld)

b=k1;

ABS = zeros(n,1);
for i=1:n
    if e(i)>0
        ABS(i) = e(i);
    else
        ABS(i) = -e(i);
    end
end
SGN = e ./ (ABS + cons_sld);

u = u1 - b*(ABS.^0.5).*SGN;

end

== matlab function Simple_4Quad_payload_10_2017a/Controllers and Observers/Cotnroller and Observer - Agent1 /Rotational #1/Differentiator/Sliding differentiator ==
  data: u output; u1 input; e input; n parameter; k1 parameter; cons_sld parameter
function u = fcn(u1,e,n,k1,cons_sld)

b=k1;

ABS = zeros(n,1);
for i=1:n
    if e(i)>0
        ABS(i) = e(i);
    else
        ABS(i) = -e(i);
    end
end
SGN = e ./ (ABS + cons_sld);

u = u1 - b*(ABS.^0.5).*SGN;

end

== matlab function Simple_4Quad_payload_10_2017a/Controllers and Observers/Controlelr and Observer - Agent3/Link #3/Differentiator/Sliding differentiator1 ==
  data: Du1 output; e input; n parameter; k2 parameter; cons_sld parameter
function Du1 = fcn(e,n,k2,cons_sld)

a=k2;

ABS = zeros(n,1);
for i=1:n
    if e(i)>0
        ABS(i) = e(i);
    else
        ABS(i) = -e(i);
    end
end
SGN = e ./ (ABS + cons_sld);

Du1 = - a*SGN;

end

== matlab function Simple_4Quad_payload_10_2017a/Controllers and Observers/Controlelr and Observer - Agent3/Link #3/g-Estimator ==
  data: sigma input; g_hat input; P input; rho_1L parameter; gamma_1L parameter; Dg_hat output
function Dg_hat = fcn(sigma,g_hat,P,rho_1L,gamma_1L)

Dg_hat = - gamma_1L * P * sigma - rho_1L * gamma_1L * g_hat;

end

== matlab function Simple_4Quad_payload_10_2017a/Controllers and Observers/Controlelr and Observer - Agent3/Link #3/g-Estimator1 ==
  data: sigma input; x input; P input; rho_0L parameter; gamma_0L parameter; Da_hat output; a_hat input
function Da_hat = fcn(sigma,x,P,rho_0L,gamma_0L,a_hat)

DVa_hat = - gamma_0L * P * diag(sigma) * (x - sigma) - rho_0L * gamma_0L * diag(a_hat);

Da_hat = diag(DVa_hat);

end

== matlab function Simple_4Quad_payload_10_2017a/Controllers and Observers/Controlelr and Observer - Agent3/Link #3/main ==
  data: sigma input; zeta input; u output; Dy_d input; R parameter; P input; a_hat input; BR parameter; g_hat input; x input; QL parameter; BBT_inv parameter; n parameter
function u = fcn(sigma,zeta,Dy_d,R,P,a_hat,BR,g_hat,x,QL,BBT_inv,n)

u1 = (1/2) * R * BR' * P * sigma;
u2 = BBT_inv * (Dy_d - a_hat*x + (eye(n) + 2*(((P)^(-1)*QL)) + a_hat)*sigma - g_hat - zeta) - (3/4) * R * BR' * P * sigma;

u = u1 + u2;

end

== matlab function Simple_4Quad_payload_10_2017a/Controllers and Observers/Controlelr and Observer - Agent3/Link #3/output definition ==
  data: u input; ur output
function ur = fcn(u)

ur = u(4:6);

end

== matlab function Simple_4Quad_payload_10_2017a/Controllers and Observers/Controlelr and Observer - Agent3/Link #3/variable change ==
  data: X input; Xd input; x_mod output; u input; xd_mod output; e_mod output
function [x_mod,xd_mod,e_mod] = fcn(X,Xd,u)

x_mod = X;

xd_mod = [Xd;u(1:3)];

e_mod = xd_mod - x_mod;


end

== matlab function Simple_4Quad_payload_10_2017a/Controllers and Observers/Cotnroller and Observer - Agent1 /Controller Interpreter #1 ==
  data: Trust1 output; ut_1 input; PHI_d_1 output; max_att parameter
function [Trust1,PHI_d_1] = fcn(ut_1,max_att)

%%
fT_1 = sqrt((ut_1(1)^2)+(ut_1(2)^2)+(ut_1(3)^2));
psi_d_1 = 0;
phi_d_1 = asin( min(max(((sin(psi_d_1)*ut_1(1) - cos(psi_d_1)*ut_1(2)) / (fT_1+0e-3)),-1),1) ); %-0.1*ut_1(2);
theta_d_1 = atan( (cos(psi_d_1)*ut_1(1) + sin(psi_d_1)*ut_1(2)) / (ut_1(3)+0e-3) ); %+0.1*ut_1(1);
PHI_d_1 = [min(max(phi_d_1,-max_att),max_att);min(max(theta_d_1,-max_att),max_att);psi_d_1]; 
Trust1 = [0;0;-fT_1];

end

== matlab function Simple_4Quad_payload_10_2017a/Controllers and Observers/Cotnroller and Observer - Agent1 /Rotational #1/Differentiator/Sliding differentiator1 ==
  data: Du1 output; e input; n parameter; k2 parameter; cons_sld parameter
function Du1 = fcn(e,n,k2,cons_sld)

a=k2;

ABS = zeros(n,1);
for i=1:n
    if e(i)>0
        ABS(i) = e(i);
    else
        ABS(i) = -e(i);
    end
end
SGN = e ./ (ABS + cons_sld);

Du1 = - a*SGN;

end

== matlab function Simple_4Quad_payload_10_2017a/Controllers and Observers/Cotnroller and Observer - Agent1 /Rotational #1/g-Estimator ==
  data: sigma input; g_hat input; P input; rho_1 parameter; gamma_1 parameter; Dg_hat output
function Dg_hat = fcn(sigma,g_hat,P,rho_1,gamma_1)

Dg_hat = - gamma_1 * P * sigma - rho_1 * gamma_1 * g_hat;

end

== matlab function Simple_4Quad_payload_10_2017a/Controllers and Observers/Cotnroller and Observer - Agent1 /Rotational #1/g-Estimator1 ==
  data: sigma input; x input; P input; rho_0 parameter; gamma_0 parameter; Da_hat output; a_hat input
function Da_hat = fcn(sigma,x,P,rho_0,gamma_0,a_hat)

DVa_hat = - gamma_0 * P * diag(sigma) * (x - sigma) - rho_0 * gamma_0 * diag(a_hat);

Da_hat = diag(DVa_hat);

end

== matlab function Simple_4Quad_payload_10_2017a/Controllers and Observers/Cotnroller and Observer - Agent1 /Rotational #1/main ==
  data: sigma input; zeta input; u output; Dy_d input; R parameter; P input; a_hat input; BR parameter; g_hat input; x input; QR parameter; BBT_inv parameter; n parameter
function u = fcn(sigma,zeta,Dy_d,R,P,a_hat,BR,g_hat,x,QR,BBT_inv,n)

u1 = (1/2) * R * BR' * P * sigma;
u2 = BBT_inv * (Dy_d - a_hat*x + (eye(n) + 2*(((P)^(-1)*QR)) + a_hat)*sigma - g_hat - zeta) - (3/4) * R * BR' * P * sigma;

u = u1 + u2;

end

== matlab function Simple_4Quad_payload_10_2017a/Controllers and Observers/Cotnroller and Observer - Agent1 /Rotational #1/variable change ==
  data: X input; Xd input; x_mod output; u input; xd_mod output; e_mod output
function [x_mod,xd_mod,e_mod] = fcn(X,Xd,u)

x_mod = X;

xd_mod = [Xd;u(1:3)];

e_mod = xd_mod - x_mod;


end

== matlab function Simple_4Quad_payload_10_2017a/Controllers and Observers/Controller and Observer - Agent4/Link #4/CARE ==
  data: P input; a_hat input; BR parameter; R parameter; DP output; QL parameter
function DP = fcn(P,a_hat,BR,R,QL)

DP = a_hat*P + P*a_hat' - P*BR*R*BR'*P + 2*QL;

end

== matlab function Simple_4Quad_payload_10_2017a/Controllers and Observers/Controller and Observer - Agent4/Link #4/Differentiator/Sliding differentiator ==
  data: u output; u1 input; e input; n parameter; k1 parameter; cons_sld parameter
function u = fcn(u1,e,n,k1,cons_sld)

b=k1;

ABS = zeros(n,1);
for i=1:n
    if e(i)>0
        ABS(i) = e(i);
    else
        ABS(i) = -e(i);
    end
end
SGN = e ./ (ABS + cons_sld);

u = u1 - b*(ABS.^0.5).*SGN;

end

== matlab function Simple_4Quad_payload_10_2017a/Controllers and Observers/Controller and Observer - Agent4/Link #4/Differentiator/Sliding differentiator1 ==
  data: Du1 output; e input; n parameter; k2 parameter; cons_sld parameter
function Du1 = fcn(e,n,k2,cons_sld)

a=k2;

ABS = zeros(n,1);
for i=1:n
    if e(i)>0
        ABS(i) = e(i);
    else
        ABS(i) = -e(i);
    end
end
SGN = e ./ (ABS + cons_sld);

Du1 = - a*SGN;

end

== matlab function Simple_4Quad_payload_10_2017a/Controllers and Observers/Controller and Observer - Agent4/Link #4/g-Estimator ==
  data: sigma input; g_hat input; P input; rho_1L parameter; gamma_1L parameter; Dg_hat output
function Dg_hat = fcn(sigma,g_hat,P,rho_1L,gamma_1L)

Dg_hat = - gamma_1L * P * sigma - rho_1L * gamma_1L * g_hat;

end

== matlab function Simple_4Quad_payload_10_2017a/Rotational Controller Log/For matrix Plot/MATLAB Function ==
  data: u input; y output
function y = fcn(u)
S1 = size(u,1);
S2 = size(u,2);

y = zeros(S1*S2,1);
num = 0;
for i=1:S1
    for j=1:S2
        num = num + 1;
        y(num,1) = u(i,j);
    end
end

end

== matlab function Simple_4Quad_payload_10_2017a/Rotational Controller Log/For matrix Plot1/MATLAB Function ==
  data: u input; y output
function y = fcn(u)
S1 = size(u,1);
S2 = size(u,2);

y = zeros(S1*S2,1);
num = 0;
for i=1:S1
    for j=1:S2
        num = num + 1;
        y(num,1) = u(i,j);
    end
end

end

== matlab function Simple_4Quad_payload_10_2017a/Rotational Controller Log/For matrix Plot2/MATLAB Function ==
  data: u input; y output
function y = fcn(u)
S1 = size(u,1);
S2 = size(u,2);

y = zeros(S1*S2,1);
num = 0;
for i=1:S1
    for j=1:S2
        num = num + 1;
        y(num,1) = u(i,j);
    end
end

end

== matlab function Simple_4Quad_payload_10_2017a/Rotational Controller Log/For matrix Plot3/MATLAB Function ==
  data: u input; y output
function y = fcn(u)
S1 = size(u,1);
S2 = size(u,2);

y = zeros(S1*S2,1);
num = 0;
for i=1:S1
    for j=1:S2
        num = num + 1;
        y(num,1) = u(i,j);
    end
end

end

== matlab function Simple_4Quad_payload_10_2017a/Rotational Controller Log/For matrix Plot4/MATLAB Function ==
  data: u input; y output
function y = fcn(u)
S1 = size(u,1);
S2 = size(u,2);

y = zeros(S1*S2,1);
num = 0;
for i=1:S1
    for j=1:S2
        num = num + 1;
        y(num,1) = u(i,j);
    end
end

end

== matlab function Simple_4Quad_payload_10_2017a/Rotational Controller Log/For matrix Plot5/MATLAB Function ==
  data: u input; y output
function y = fcn(u)
S1 = size(u,1);
S2 = size(u,2);

y = zeros(S1*S2,1);
num = 0;
for i=1:S1
    for j=1:S2
        num = num + 1;
        y(num,1) = u(i,j);
    end
end

end

== matlab function Simple_4Quad_payload_10_2017a/Controllers and Observers/Controller and Observer - Agent4/Link #4/g-Estimator1 ==
  data: sigma input; x input; P input; rho_0L parameter; gamma_0L parameter; Da_hat output; a_hat input
function Da_hat = fcn(sigma,x,P,rho_0L,gamma_0L,a_hat)

DVa_hat = - gamma_0L * P * diag(sigma) * (x - sigma) - rho_0L * gamma_0L * diag(a_hat);

Da_hat = diag(DVa_hat);

end

== matlab function Simple_4Quad_payload_10_2017a/Controllers and Observers/Controller and Observer - Agent4/Link #4/main ==
  data: sigma input; zeta input; u output; Dy_d input; R parameter; P input; a_hat input; BR parameter; g_hat input; x input; QL parameter; BBT_inv parameter; n parameter
function u = fcn(sigma,zeta,Dy_d,R,P,a_hat,BR,g_hat,x,QL,BBT_inv,n)

u1 = (1/2) * R * BR' * P * sigma;
u2 = BBT_inv * (Dy_d - a_hat*x + (eye(n) + 2*(((P)^(-1)*QL)) + a_hat)*sigma - g_hat - zeta) - (3/4) * R * BR' * P * sigma;

u = u1 + u2;

end

== matlab function Simple_4Quad_payload_10_2017a/Controllers and Observers/Controller and Observer - Agent4/Link #4/output definition ==
  data: u input; ur output
function ur = fcn(u)

ur = u(4:6);

end

== matlab function Simple_4Quad_payload_10_2017a/Controllers and Observers/Controller and Observer - Agent4/Link #4/variable change ==
  data: X input; Xd input; x_mod output; u input; xd_mod output; e_mod output
function [x_mod,xd_mod,e_mod] = fcn(X,Xd,u)

x_mod = X;

xd_mod = [Xd;u(1:3)];

e_mod = xd_mod - x_mod;


end

== matlab function Simple_4Quad_payload_10_2017a/Controllers and Observers/Controller - Payload/Payload_pos/CARE ==
  data: P input; a_hat input; BRp parameter; Rp parameter; DP output; Qp parameter
function DP = fcn(P,a_hat,BRp,Rp,Qp)

DP = a_hat*P + P*a_hat' - P*BRp*Rp*BRp'*P + 2*Qp;

end

== matlab function Simple_4Quad_payload_10_2017a/Rotational Controller Log/For matrix Plot6/MATLAB Function ==
  data: u input; y output
function y = fcn(u)
S1 = size(u,1);
S2 = size(u,2);

y = zeros(S1*S2,1);
num = 0;
for i=1:S1
    for j=1:S2
        num = num + 1;
        y(num,1) = u(i,j);
    end
end

end

== matlab function Simple_4Quad_payload_10_2017a/Controllers and Observers/Controller - Payload/Payload_pos/Differentiator/Sliding differentiator ==
  data: u output; u1 input; e input; np parameter; k1 parameter; alpha_chatt parameter
function u = fcn(u1,e,np,k1,alpha_chatt)

b=k1;

ABS = zeros(np,1);
for i=1:np
    if e(i)>0
        ABS(i) = e(i);
    else
        ABS(i) = -e(i);
    end
end
SGN = e ./ (ABS + alpha_chatt);

u = u1 - b*(ABS.^0.5).*SGN;

end

== matlab function Simple_4Quad_payload_10_2017a/Rotational Controller Log/For matrix Plot7/MATLAB Function ==
  data: u input; y output
function y = fcn(u)
S1 = size(u,1);
S2 = size(u,2);

y = zeros(S1*S2,1);
num = 0;
for i=1:S1
    for j=1:S2
        num = num + 1;
        y(num,1) = u(i,j);
    end
end

end

== matlab function Simple_4Quad_payload_10_2017a/Controllers and Observers/Controller - Payload/Payload_pos/Differentiator/Sliding differentiator1 ==
  data: Du1 output; e input; np parameter; k2 parameter; alpha_chatt parameter
function Du1 = fcn(e,np,k2,alpha_chatt)

a=k2;

ABS = zeros(np,1);
for i=1:np
    if e(i)>0
        ABS(i) = e(i);
    else
        ABS(i) = -e(i);
    end
end
SGN = e ./ (ABS + alpha_chatt);

Du1 = - a*SGN;

end

== matlab function Simple_4Quad_payload_10_2017a/Controllers and Observers/Controller - Payload/Payload_pos/g-Estimator ==
  data: sigma input; g_hat input; P input; rho_1p parameter; gamma_1p parameter; Dg_hat output
function Dg_hat = fcn(sigma,g_hat,P,rho_1p,gamma_1p)

Dg_hat = - gamma_1p * P * sigma - rho_1p * gamma_1p * g_hat;

end

== matlab function Simple_4Quad_payload_10_2017a/Controllers and Observers/Controller - Payload/Payload_pos/g-Estimator1 ==
  data: sigma input; x input; P input; rho_0p parameter; gamma_0p parameter; Da_hat output; a_hat input
function Da_hat = fcn(sigma,x,P,rho_0p,gamma_0p,a_hat)

DVa_hat = - gamma_0p * P * diag(sigma) * (x - sigma) - rho_0p * gamma_0p * diag(a_hat);

Da_hat = diag(DVa_hat);

end

== matlab function Simple_4Quad_payload_10_2017a/Controllers and Observers/Controller - Payload/Payload_pos/main ==
  data: sigma input; zeta input; u output; Dy_d input; Rp parameter; P input; a_hat input; BRp parameter; g_hat input; x input; Qp parameter; BBT_invp parameter; np parameter
function u = fcn(sigma,zeta,Dy_d,Rp,P,a_hat,BRp,g_hat,x,Qp,BBT_invp,np)

u1 = (1/2) * Rp * BRp' * P * sigma;
u2 = BBT_invp * (Dy_d - a_hat*x + (eye(np) + 2*(((P)^(-1)*Qp)) + a_hat)*sigma - g_hat - zeta) - (3/4) * Rp * BRp' * P * sigma;

u = u1 + u2;

end

== matlab function Simple_4Quad_payload_10_2017a/Controllers and Observers/Controller - Payload/Payload_vel/CARE ==
  data: P input; a_hat input; BRp parameter; Rp parameter; DP output; Qv parameter
function DP = fcn(P,a_hat,BRp,Rp,Qv)

DP = a_hat*P + P*a_hat' - P*BRp*Rp*BRp'*P + 2*Qv;

end

== matlab function Simple_4Quad_payload_10_2017a/Controllers and Observers/Controller - Payload/Payload_pos/variable change ==
  data: X input; Xd input; x_mod output; xd_mod output; e_mod output
function [x_mod,xd_mod,e_mod] = fcn(X,Xd)

x_mod = X;

xd_mod = Xd;

e_mod = xd_mod - x_mod;


end

== matlab function Simple_4Quad_payload_10_2017a/Controllers and Observers/Controller - Payload/Payload_vel/Differentiator/Sliding differentiator ==
  data: u output; u1 input; e input; np parameter; k1 parameter; alpha_chatt parameter
function u = fcn(u1,e,np,k1,alpha_chatt)

b=k1;

ABS = zeros(np,1);
for i=1:np
    if e(i)>0
        ABS(i) = e(i);
    else
        ABS(i) = -e(i);
    end
end
SGN = e ./ (ABS + alpha_chatt);

u = u1 - b*(ABS.^0.5).*SGN;

end

== matlab function Simple_4Quad_payload_10_2017a/Controllers and Observers/Controller - Payload/Payload_vel/Differentiator/Sliding differentiator1 ==
  data: Du1 output; e input; np parameter; k2 parameter; alpha_chatt parameter
function Du1 = fcn(e,np,k2,alpha_chatt)

a=k2;

ABS = zeros(np,1);
for i=1:np
    if e(i)>0
        ABS(i) = e(i);
    else
        ABS(i) = -e(i);
    end
end
SGN = e ./ (ABS + alpha_chatt);

Du1 = - a*SGN;

end

== matlab function Simple_4Quad_payload_10_2017a/Controllers and Observers/Controller - Payload/Payload_vel/g-Estimator ==
  data: sigma input; g_hat input; P input; rho_1v parameter; gamma_1v parameter; Dg_hat output
function Dg_hat = fcn(sigma,g_hat,P,rho_1v,gamma_1v)

Dg_hat = - gamma_1v * P * sigma - rho_1v * gamma_1v * g_hat;

end
